simulink model "rtwdemo_comments"  (Simulink 7.6)
settings: Solver=FixedStepDiscrete  SolverMode=SingleTasking  StartTime=0.0  StopTime=10  FixedStep=0.001  RelTol=1e-3  SampleTimeConstraint=STIndependent
PreLoadFcn:
  | rtwdemo_comments_data;
values from neighbouring files (symbols this model uses):
  const_val = Simulink.Parameter    [rtwdemo_comments_data.m]
libraries: simulink x1
Description:
  | User-Controlled Comments to Improve Code Readability and Traceability
settings Model: Creator=The MathWorks Inc.  ExtModeAutoUpdateStatusClock=off
settings MATStruct: SampleTime=0.001  Offset=0  Priority=[20.0]
settings DataIOCC: ExternalInput=[tim_var, data_var]  SaveOutput=off  SaveTime=off
settings OptimizationCC: InlineParams=on  InlineInvariantSignals=on  PassReuseOutputArgsAs=Individual arguments  StateBitsets=on  DataBitsets=on  UseTempVars=on  ZeroExternalMemoryAtStartup=off  ZeroInternalMemoryAtStartup=off  NoFixptDivByZeroProtection=on  EfficientFloat2IntCast=on  EfficientMapNaN2IntZero=off  OptimizeModelRefInitCode=on  LifeSpan=1  BufferReusableBoundary=off
settings DebuggingCC: CheckExecutionContextPreStartOutputMsg=on  CheckExecutionContextRuntimeOutputMsg=on  SolverPrmCheckMsg=none  SigSpecEnsureSampleTimeMsg=none  StrictBusMsg=ErrorOnBusTreatedAsVector
settings HardwareCC: ProdIntDivRoundTo=Zero  ProdEndianess=LittleEndian  ProdHWDeviceType=Generic->32-bit Embedded Processor  TargetHWDeviceType=Generic->32-bit Embedded Processor
settings SFSimCC: SimParseCustomCode=off
settings RTWCC: SystemTargetFile=ert.tlc  TLCOptions=-p0 -aWarnNonSaturatedBlocks=0  TemplateMakefile=ert_default_tmf  Description=Real-Time Workshop Embedded Coder (no auto configuration)  GenerateReport=on  RTWVerbose=off  ProcessScript=ert_make_rtw_hook  IncludeHyperlinkInReport=on  LaunchReport=on
settings CodeAppCC: ForceParamTrailComments=on  IgnoreCustomStorageClasses=off  IgnoreTestpoints=on  SimulinkDataObjDesc=on  SFDataObjDesc=on  CustomSymbolStrGlobalVar=rt$N$M  CustomSymbolStrFcn=$F$N$M  CustomSymbolStrMacro=$N$M  CustomCommentsFcn=rtwdemo_comments_mptfun.m  InsertBlockDesc=on  EnableCustomComments=on
settings ERTTargetCC: TargetFcnLib=ansi_tfl_tmw.mat  MultiwordLength=2048  GenerateSampleERTMain=on  IncludeMdlTerminateFcn=off  SupportNonFinite=off  SupportComplex=off  InlinedParameterPlacement=NonHierarchical  ERTSrcFileBannerTemplate=rtwdemo_comments.cgt  ERTHdrFileBannerTemplate=rtwdemo_comments.cgt  ERTDataSrcFileTemplate=rtwdemo_comments.cgt  ERTDataHdrFileTemplate=rtwdemo_comments.cgt  ERTCustomFileTemplate=example_file_process.tlc  ConvertIfToSwitch=off

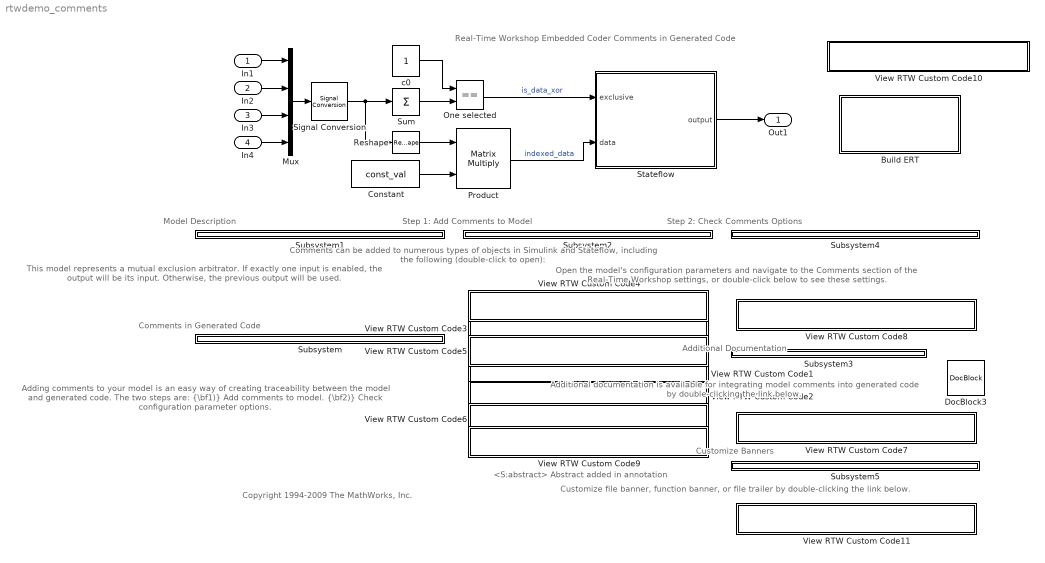
== system rtwdemo_comments ==
  note: This model represents a mutual exclusion
      | arbitrator.  If exactly one input is enabled,
      | the output will be its input.  Otherwise,
      | the previous output will be used.
  note: Real-Time Workshop Embedded Coder
      | Comments in Generated Code
  note: Comments in Generated Code
  note: Adding comments to your model is an easy
      | way of creating traceability between the model
      | and generated code.  The two steps are:
      |
      |   {\bf1)} Add comments to model.
      |   {\bf2)} Check configuration parameter options.
  note: Additional Documentation
  note: Additional documentation is available
      | for integrating model comments into
      | generated code by double-clicking the
      | link below.
  note: Comments can be added to numerous types
      | of objects in Simulink and Stateflow, including
      | the following (double-click to open):
  note: Model Description
  note: Open the model's configuration parameters
      | and navigate to the Comments section of
      | the Real-Time Workshop settings, or
      | double-click below to see these settings.
  note: Step 1: Add Comments to Model
  note: Step 2: Check Comments Options
  note: <S:abstract> Abstract added in annotation
  note: Copyright 1994-2009 The MathWorks, Inc.
  note: Customize Banners
  note: Customize file banner, function banner,
      | or file trailer by double-clicking the link below.
  In1 : Inport  OutDataTypeStr=double  PortDimensions=1
  In2 : Inport  Port=2  OutDataTypeStr=double  PortDimensions=1
  In3 : Inport  Port=3  OutDataTypeStr=double  PortDimensions=1
  In4 : Inport  Port=4  OutDataTypeStr=double  PortDimensions=1
  Build ERT : Subsystem  mask{attrib_overrides={'ERTSrcFileBannerTemplate','ERTHdrFileBannerTemplate','ERTDataSrcFileTemplate','ERTDataHdrFileTemplate'}}
      mask prompts: attrib_overrides "List of attributes to preserve (cell of strings):"
      mask help: Enter the attributes of the configuration set that you want preserved. Otherwise, the default configuration script will override your current settings.
      settings: OpenFcn=|
      | model=bdroot; overrides=get_param(gcb,'attrib_overrides');
      | try
      | 
      | set_param(model,'LoadExternalInput','off')
      | rtwconfiguredemo(model,'noop',false,overrides);
      | rtwbuilddemomodel(model);
      | set_param(model,'LoadExternalInput','on')
      | set_param(model,'dirty','off')
      | 
      | catch
      |   error(lasterr);
      | end
      |                        clear model overrides;
      mask Display:
      | disp(['Generate Code Using\n',...
      | 	  'Real-Time Workshop\n',...
      | 	  'Embedded Coder\n'...
      | 	  '(double-click)'])
  Constant : Constant  Value=const_val  VectorParams1D=off  OutDataTypeStr=double
  DocBlock3 : simulink/Model-Wide Utilities/DocBlock  SystemSampleTime=-1  ECoderFlag=History  DocumentType=Text
      settings: AttributesFormatString=%<ECoderFlag>
  Mux : Mux
  "One selected " : RelationalOperator  Description=This block determines if exactly one input is enabled.  Operator===  OutDataTypeStr=boolean
  Product : Product  Description=This block determines the output index by taking the inner product of the vector of inputs and [1 2 3 4].  Multiplication=Matrix(*)  OutDataTypeStr=double  RndMeth=Zero
  Reshape : Reshape  OutputDimensionality=Row vector (2-D)
  Signal Conversion : SignalConversion  ConversionOutput=Contiguous copy  OverrideOpt=on
  Stateflow : Stateflow chart  Description=|  TreatAsAtomicUnit=on
      | Stateflow block decides the index output by following logic   
      | 1. If one and only one input signal is enabled, the index will
      | refer to the enabled signal line.                             
      | 2. Otherwise, maintain the old value.
  Subsystem : Subsystem
  Subsystem1 : Subsystem
  Subsystem2 : Subsystem
  Subsystem3 : Subsystem
  Subsystem4 : Subsystem
  Subsystem5 : Subsystem
  Sum : Sum  Description=This block counts the number of enabled inputs.  Inputs=+  OutDataTypeStr=double  InputSameDT=on
  View RTW Custom Code1 : Subsystem
      mask init:
      | pos    = get_param(gcb, 'Position');
      | width  = pos(3) - pos(1);
      | height = pos(4) - pos(2);
      | 
      | 
      | % Compute arrow coordinates
      | arrowW = width  / 20;
      | arrowH = height / 2.5;
      | arrowX = width  / 50;
      | arrowY = height / 3;
      | arrowXvec = [arrowX, arrowX, arrowX + arrowW];
      | arrowYvec = [arrowY, arrowY + arrowH, arrowY + arrowH / 2];
      | 
      | % Compute text position
      | textXbuff = width / 30;
      | textX  = arrowX + arrowW + textXbuff;
      | textY  = height / 2;
      settings: OpenFcn=|
      | y = DAStudio.Dialog(is_data_xor);
      | y.setTitle('Simulink.Signal: is_data_xor'); clear y;
      mask Display:
      | patch(arrowXvec, arrowYvec);
      | text(textX, textY, 'Simulink Signal Object');
  View RTW Custom Code10 : Subsystem
      mask init: same as rtwdemo_comments/View RTW Custom Code1
      settings: OpenFcn=|
      | currentEncSetting = slCharacterEncoding;
      | if ~strcmp(currentEncSetting,'ibm-943_P14A-2000') && ...
      |         ~strcmp(currentEncSetting,'Shift_JIS')
      |     warndlg('The current Simulink character encoding setting does not match the demo model character encoding. You must change the current character encoding to "Shift_JIS" to load the model. Type "help slCharacterEncoding" for more information.');
      | else
      |     rtwdemo_international;
      | end;                    clear currentEncSetting;
      mask Display:
      | patch(arrowXvec, arrowYvec);
      | text(textX, textY, 'Open International Demo');
  View RTW Custom Code11 : Subsystem
      mask init: same as rtwdemo_comments/View RTW Custom Code1
      settings: OpenFcn=edit rtwdemo_comments.cgt
      mask Display:
      | patch(arrowXvec, arrowYvec);
      | text(textX, textY, 'Customize banners via code templates');
  View RTW Custom Code2 : Subsystem
      mask init: same as rtwdemo_comments/View RTW Custom Code1
      settings: OpenFcn=|
      | y = DAStudio.Dialog(const_val);
      | y.setTitle('Simulink.Parameter: const_val'); clear y;
      mask Display:
      | patch(arrowXvec, arrowYvec);
      | text(textX, textY, 'Simulink Parameter Object');
  View RTW Custom Code3 : Subsystem
      mask init: same as rtwdemo_comments/View RTW Custom Code1
      settings: OpenFcn=|
      | state=find(sfroot,'-isa','Stateflow.State','-and','Name','Normal');
      | sf('Open',state.id);
      | dlg = DAStudio.Dialog(state);   clear state dlg;
      mask Display:
      | patch(arrowXvec, arrowYvec);
      | text(textX, textY, 'Stateflow State');
  View RTW Custom Code4 : Subsystem
      mask init: same as rtwdemo_comments/View RTW Custom Code1
      settings: OpenFcn=|
      | block=[bdroot, '/Product'];
      | hilite_system(block);
      | open_system(block, 'property'); clear block;
      mask Display:
      | patch(arrowXvec, arrowYvec);
      | text(textX, textY, 'Simulink Block');
  View RTW Custom Code5 : Subsystem
      mask init: same as rtwdemo_comments/View RTW Custom Code1
      settings: OpenFcn=|
      | trans=find(sfroot,'-isa','Stateflow.Transition','-and','LabelString','// After initialize');
      | sf('Open',trans.id);
      | dlg = DAStudio.Dialog(trans);  clear trans dlg;
      mask Display:
      | patch(arrowXvec, arrowYvec);
      | text(textX, textY, 'Stateflow Transition');
  View RTW Custom Code6 : Subsystem
      mask init: same as rtwdemo_comments/View RTW Custom Code1
      settings: OpenFcn=|
      | y = DAStudio.Dialog(indexed_data);
      | y.setTitle('mpt.Signal: indexed_data'); clear y;
      mask Display:
      | patch(arrowXvec, arrowYvec);
      | text(textX, textY, 'MPT Signal Object');
  View RTW Custom Code7 : Subsystem
      mask init: same as rtwdemo_comments/View RTW Custom Code1
      settings: OpenFcn=helpview([docroot '/toolbox/ecoder/helptargets.map'], 'ecoder_comments_pane')
      mask Display:
      | patch(arrowXvec, arrowYvec);
      | text(textX, textY, 'Comments Documentation');
  View RTW Custom Code8 : Subsystem
      mask init: same as rtwdemo_comments/View RTW Custom Code1
      settings: OpenFcn=|
      | model = bdroot;
      | dlg = slCfgPrmDlg(model,'Open');
      | dlg = slCfgPrmDlg(bdroot,'TurnToPage','Comments'); clear model dlg;
      mask Display:
      | patch(arrowXvec, arrowYvec);
      | text(textX, textY, 'Open Comments Settings');
  View RTW Custom Code9 : Subsystem
      mask init: same as rtwdemo_comments/View RTW Custom Code1
      settings: OpenFcn=edit rtwdemo_comments_mptfun.m;
      mask Display:
      | patch(arrowXvec, arrowYvec);
      | text(textX, textY, 'MPT Callback Function');
  c0 : Constant
  Out1 : Outport
  wires:
  Mux/1 -> Signal Conversion/1
  Constant/1 -> Product/2
  c0/1 -> "One selected "/1
  Sum/1 -> "One selected "/2
  "One selected "/1 -> Stateflow/1(exclusive)  "is_data_xor"
  Product/1 -> Stateflow/2(data)  "indexed_data"
  Stateflow/1(output) -> Out1/1
  In1/1 -> Mux/1
  In2/1 -> Mux/2
  In3/1 -> Mux/3
  In4/1 -> Mux/4
  Signal Conversion/1 -> Sum/1, Reshape/1
  Reshape/1 -> Product/1

== system rtwdemo_comments/Build ERT ==

== system rtwdemo_comments/Subsystem ==

== system rtwdemo_comments/Subsystem1 ==

== system rtwdemo_comments/Subsystem2 ==

== system rtwdemo_comments/Subsystem3 ==

== system rtwdemo_comments/Subsystem4 ==

== system rtwdemo_comments/Subsystem5 ==

== system rtwdemo_comments/View RTW Custom Code1 ==

== system rtwdemo_comments/View RTW Custom Code10 ==

== system rtwdemo_comments/View RTW Custom Code11 ==

== system rtwdemo_comments/View RTW Custom Code2 ==

== system rtwdemo_comments/View RTW Custom Code3 ==

== system rtwdemo_comments/View RTW Custom Code4 ==

== system rtwdemo_comments/View RTW Custom Code5 ==

== system rtwdemo_comments/View RTW Custom Code6 ==

== system rtwdemo_comments/View RTW Custom Code7 ==

== system rtwdemo_comments/View RTW Custom Code8 ==

== system rtwdemo_comments/View RTW Custom Code9 ==

== stateflow chart Stateflow ==
  state Normal
    settings: description=This state determines the value of the output after the intialization.
    (default) -> (junction 6)
    (junction 6) -> (junction 7) [order 1] : [exclusive]
      settings: description=This transition is taken when exactly one input is enabled.
    (junction 7) -> (junction 8) : {output=data;}
      settings: description=This transition assigns the output to the index of the only enabled input.
    (junction 8) -> (junction 9)
    (junction 6) -> (junction 9) [order 2] : // Output has
        | // previous value
    Normal -> (junction 6)
  state First
    entry: output=1;
    settings: description=The state is activated at initialization.
  note: <S:Description> Description added in Stateflow note
  (default) -> First
  First -> Normal : // After initialize
    settings: description=After initialization, transfer to the normal state.
  data: exclusive input boolean; data input double; output output int32
